simulink model "delay"  (R2020a)
settings: Solver=FixedStepDiscrete  StartTime=0.0  StopTime=inf  RelTol=1e-3
libraries: dspsnks4 x1, dspvision x1
settings Model: Creator=unity  LastModifiedBy=unity
settings SolverCC: AutoInsertRateTranBlk=on
settings DataIOCC: LimitDataPoints=on  SaveOutput=off  SignalLogging=off  SaveTime=off
settings OptimizationCC: LifeSpan=inf
settings DebuggingCC: AlgebraicLoopMsg=error  SingleTaskRateTransMsg=error  AllowSymbolicDim=off  SFUnexpectedBacktrackingDiag=warning  SFNoUnconditionalDefaultTransitionDiag=warning  SFExecutionAtInitializationDiag=none  ArithmeticOperatorsInVariantConditions=warning
settings SFSimCC: SimUseLocalCustomCode=off  CustomCodeUndefinedFunction=UseInterfaceOnly
settings RTWCC: RTWUseLocalCustomCode=off
settings CodeAppCC: StateflowObjectComments=on
settings GRTTargetCC: TargetLangStandard=C89/C90 (ANSI)
settings ConfigComp: CovMetricSettings=dw  CovHtmlReporting=on  CovSaveCumulativeToWorkspaceVar=on  CovSaveSingleToWorkspaceVar=on  CovExternalEMLEnable=off  CovSFcnEnable=off

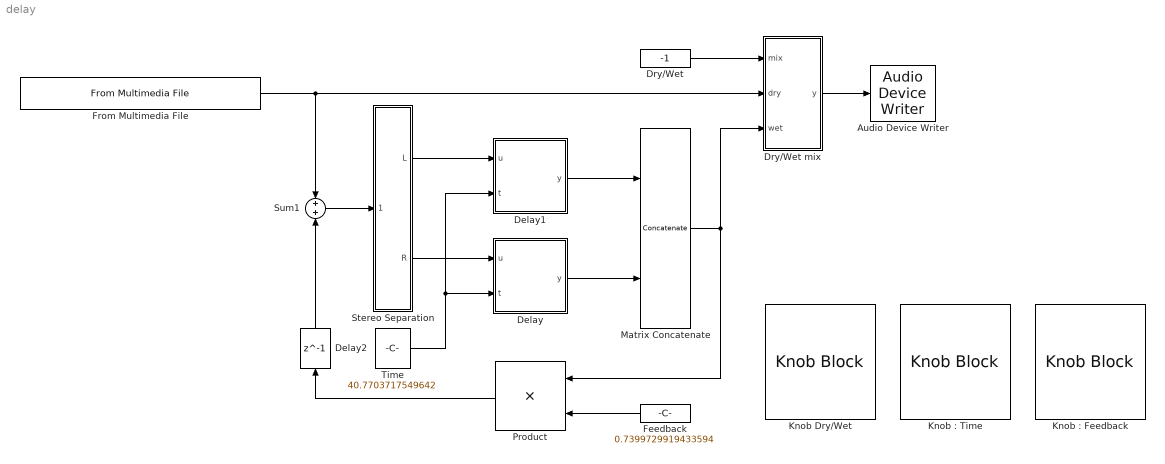
== system delay ==
  Audio Device Writer : dspsnks4/Audio Device Writer  Driver=DirectSound  Device=Default  InheritSampleRate=on  SampleRate=44100  BitDepth=16-bit integer  BufferSize=4096  NumBuffers=10  DefaultOutputChannelMapping=on  OutputChannelMapping=1:2  OutputNumUnderrunSamples=off  DriverIdx=1  DeviceWarnFlag=''
  Delay : MATLAB Function  TreatAsAtomicUnit=on
  Delay1 : MATLAB Function  TreatAsAtomicUnit=on
  Delay2 : Delay  DelayLength=1  InitialCondition=0
  Dry/Wet : Constant  Value=-1
  Dry/Wet mix : MATLAB Function  TreatAsAtomicUnit=on
  Feedback : Constant  Value=0.7399729919433594
  From Multimedia File : dspvision/From Multimedia File  inputFilename=D:\Program Files\MATLAB\R2020a\toolbox\audio\samples\FunkyDrums-44p1-stereo-25secs.mp3  readRange=[1 Inf]  loop=on  numPlays=inf  outputStreams=オーディオのみ  videoDataType=single  audioDataType=double  inheritSampleTime=on  userDefinedSampleTime=1/30  noAudioOutput=off  isIntensityVideo=off  fourcc=RGB  colorVideoFormat=Separate color signals  outputEOF=off  dataOrg=Column-major  audioFrameSize=1024  computeAudioFrameSize=off  outSamplingMode=Sample based
  "Knob : Feedback" : KnobBlock  LabelPosition=Hide  ScaleMax=1
  "Knob : Time" : KnobBlock  LabelPosition=Hide  ScaleMax=10000
  Knob Dry/Wet : KnobBlock  LabelPosition=Hide  ScaleMin=-1  ScaleMax=1
  Matrix Concatenate : Concatenate  Mode=Multidimensional array  ConcatenateDimension=2
  Product : Product
  Stereo Separation : MATLAB Function  TreatAsAtomicUnit=on
  Sum1 : Sum  Inputs=+|+
  Time : Constant  Value=40.7703717549642  OutDataTypeStr=int32
  wires:
  Time/1 -> Delay1/2(t), Delay/2(t)
  From Multimedia File/1 -> Sum1/1, Dry/Wet mix/2(dry)
  Stereo Separation/2(R) -> Delay/1(u)
  Delay/1(y) -> Matrix Concatenate/2
  Delay1/1(y) -> Matrix Concatenate/1
  Dry/Wet mix/1(y) -> Audio Device Writer/1
  Sum1/1 -> Stereo Separation/1(Stereo)
  Matrix Concatenate/1 -> Dry/Wet mix/3(wet), Product/1
  Feedback/1 -> Product/2
  Delay2/1 -> Sum1/2
  Product/1 -> Delay2/1
  Stereo Separation/1(L) -> Delay1/1(u)
  Dry/Wet/1 -> Dry/Wet mix/1(mix)

== matlab function delay/Delay ==
  data: u input; y output; t input
function y = fcn(u,t)
    frame = length(u);
    bfsize = 100000;
    persistent buffer
    if isempty(buffer)
        buffer=zeros(bfsize,1);
    end
    
    buffer(frame+1:end)=buffer(1:end-frame);
    buffer(1:frame)=flip(u);
    
y = flip(buffer(t+1:t+frame));

== matlab function delay/Stereo Separation ==
  data: Stereo input; L output; R output
function [L,R] = stat(Stereo)
    L = Stereo(:,1);
    R = Stereo(:,2);
end

== matlab function delay/Delay1 ==
  data: u input; y output; t input
function y = fcn(u,t)
    frame = length(u);
    bfsize = 100000;
    persistent buffer
    if isempty(buffer)
        buffer=zeros(bfsize,1);
    end
    
    buffer(frame+1:end)=buffer(1:end-frame);
    buffer(1:frame)=flip(u);
    
y = flip(buffer(t+1:t+frame));

== matlab function delay/Dry//Wet mix ==
  data: mix input; dry input; y output; wet input
function y = fcn(mix,dry,wet)
y = dry*min(-mix+1,1)+wet*min(mix+1,1);
